simulink model "Test_Model_HR12_2016"  (R2016b)
settings: Solver=FixedStepAuto  StartTime=0.0  StopTime=length(ipoint)  FixedStep=dt  RelTol=1e-3
values from neighbouring files (symbols this model uses):
  Cbx_cyl_fill_efy_intk_mfld_prs_atm_prs_cor_cho = true    [Calib_mdl_RSA.m]
  Cbx_cyl_fill_efy_opt_cho = false    [Calib_mdl_RSA.m]
  Cbx_cyl_fill_igr_opt_cho = false    [Calib_mdl_RSA.m]
  Cbx_ex_vvt_conf = true    [Calib_mdl_RSA.m]
  Cnx_cyl_fill_ex_mfld_prs_cor_cho = 0    [Cal_basic.m]
  Cnx_cyl_nr_conf = 3    [Cal_basic.m]
  Cxx_cyl_fill_efy_drv_max = 20    [Calib_mdl_RSA.m]
  Cxx_cyl_fill_efy_dyn_max = 0.15    [Calib_mdl_RSA.m]
  Cxx_cyl_fill_efy_dyn_min = 0    [Calib_mdl_RSA.m]
  Cxx_cyl_fill_efy_dz = 0.45    [Calib_mdl_RSA.m]
  Cxx_cyl_fill_efy_ovlp_angl = 66    [Calib_mdl_RSA.m]
  Cxx_cyl_fill_efy_vvt_ofs = 0    [Calib_mdl_RSA.m]
  Cxx_cyl_fill_trap_area_h_thd = 0.2    [Cal_basic.m]
  Cxx_cyl_fill_trap_area_l_thd = 0.1    [Cal_basic.m]
  Cxx_cyl_fill_trap_efy_dz_l_thd = 1    [Cal_basic.m]
  Cxx_cyl_fill_trap_efy_dz_neg_slop = -0.5    [Cal_basic.m]
  Cxx_cyl_fill_trap_efy_dz_pos_slop = 0.5    [Cal_basic.m]
  Cxx_cyl_fill_trap_vvt_ovlp_angl = 120    [Calib_mdl_RSA.m]
  Cxx_cyl_vol = 3.9961e-04*3    (= 0.00119883)    [Cal_basic.m]    (also in Calib_mdl_RSA.m = 0.00119900004938)
  Cxx_min_cyl_fill_mdl_ex_mfld_prs_rat_cor = 0    [Cal_basic.m]
  Nnx_eng_run_stt = 2    [Calib_mdl_RSA.m]
  Nxx_atm_kpa = 101.3    [Cal_basic.m]
  Nxx_k_degc = 273.15    [Cal_basic.m]
  Nxx_kilo_bas = 1000    [Cal_basic.m]
  Nxx_wht_pgc_j_kg = 287    [Cal_basic.m]
undefined symbols (not defined in the file or in its folder): Cxx_egr_spc_heat, Cxx_thr_spc_heat, docblock, MapFilling_Aspirated
libraries: AEMS_Standard_Library x78, simulink x2
(part 5 of 5)

== matlab function Test_Model_HR12_2016/ASXX_MWIN_TMP/ASXX_MWIN_TMP_ivlvtmd_20ms/B2_INTK_VLV_TEMP/Embedded MATLAB Function2 ==
  data: Tman input; Tco input; Tvlv output; QA input
function Tvlv=f_Tvlv(Tman, Tco, QA)

y = [0.100000001490116,0.0649999976158142,0.0500000007450581,0.0350000001490116,0.0299999993294478,0.0299999993294478,0.0250000003725290,0.0250000003725290,0.0250000003725290,0.0250000003725290,0.0250000003725290,0.0250000003725290,0.0250000003725290,0.0250000003725290,0.0250000003725290,0.0250000003725290];
x = [0,12,24,36,48,60,72,84,96,108,120,132,144,156,168,180];

Tvlv = (Tman-Tco).*interp1(x,y,QA)+Tman;
